simulink subsystem "BalanceLimit"  (R2023b)
settings: Solver=VariableStepAuto  StartTime=0.0  StopTime=10.0  RelTol=1e-3
libraries: simulink x1
settings Model: Creator=Veimar  LastModifiedBy=Veimar

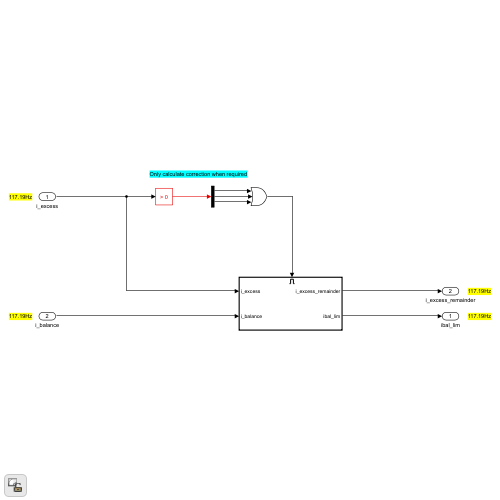
[thumbnail: Simulink's stored preview of the top-level diagram]
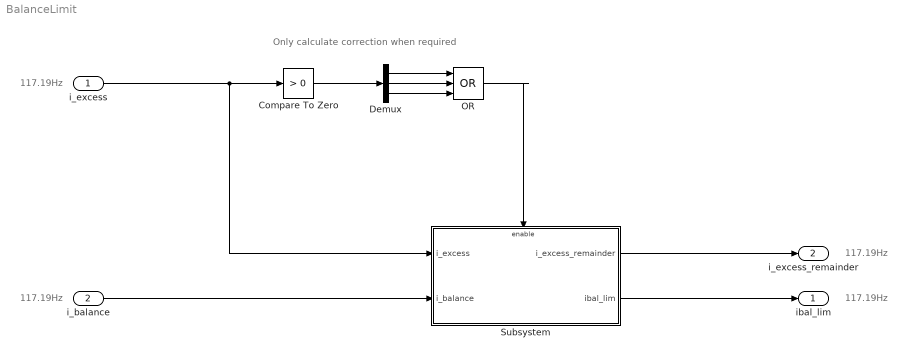
== system BalanceLimit ==
  note: Only calculate correction when required
  note: 117.19Hz
  note: 117.19Hz
  note: 117.19Hz
  note: 117.19Hz
  i_excess : Inport  OutDataTypeStr=single  PortDimensions=3
  i_balance : Inport  Port=2  OutDataTypeStr=single  PortDimensions=3
  Compare To Zero : simulink/Logic and Bit Operations/Compare To Zero  relop=>  OutDataTypeStr=boolean
  Demux : Demux  Outputs=3
  OR : Logic  Operator=OR  Inputs=3  IconShape=distinctive  AllPortsSameDT=off  OutDataTypeStr=boolean
  Subsystem : Subsystem
  ibal_lim : Outport  OutDataTypeStr=single  PortDimensions=3
  i_excess_remainder : Outport  Port=2  OutDataTypeStr=single  PortDimensions=3
  wires:
  OR/1 -> Subsystem/Enable
  Demux/3 -> OR/3
  Demux/2 -> OR/2
  Demux/1 -> OR/1
  Compare To Zero/1 -> Demux/1
  i_excess/1 -> Compare To Zero/1, Subsystem/1(i_excess)
  i_balance/1 -> Subsystem/2(i_balance)
  Subsystem/1(i_excess_remainder) -> i_excess_remainder/1
  Subsystem/2(ibal_lim) -> ibal_lim/1

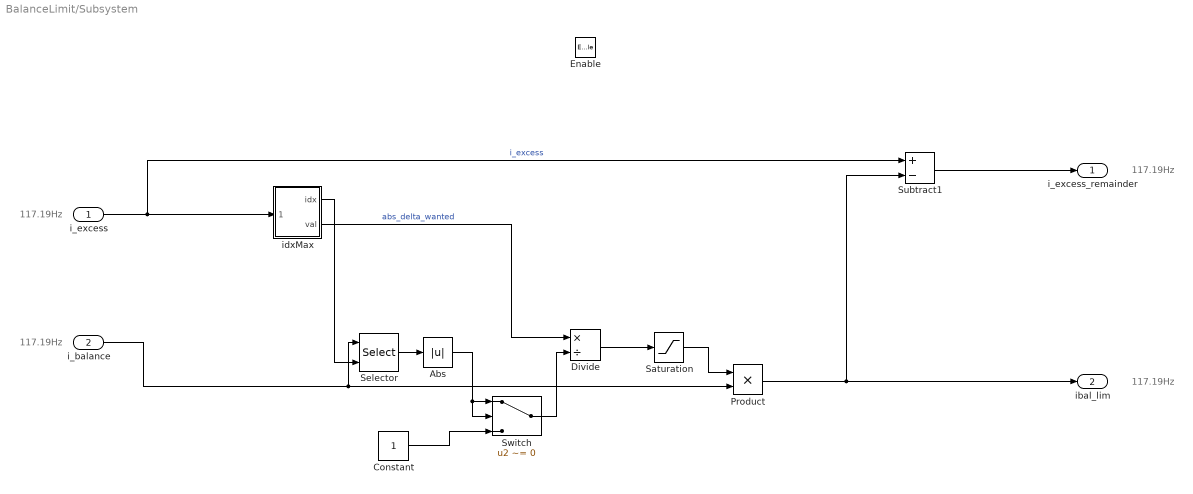
== system BalanceLimit/Subsystem ==
  note: 117.19Hz
  note: 117.19Hz
  note: 117.19Hz
  note: 117.19Hz
  i_excess : Inport
  i_balance : Inport  Port=2
  Enable : EnablePort  StatesWhenEnabling=reset
  Abs : Abs  SaturateOnIntegerOverflow=off
  Constant : Constant  OutDataTypeStr=single
  Divide : Product  Inputs=*/
  Product : Product
  Saturation : Saturate  UpperLimit=1  LowerLimit=0
  Selector : Selector  InputPortWidth=3  IndexOptions=Index vector (port)  Indices=[1 3]  OutputSizes=1
  Subtract1 : Sum  Inputs=+-
  Switch : Switch  Criteria=u2 ~= 0  SaturateOnIntegerOverflow=off  InputSameDT=off
  idxMax : Subsystem  mask(idxMinMax){maskOp=Max}
      mask prompts: maskOp "Operator"
      mask help:
      | <html><p>
      | The idxMinMax block determines the minimum or maximum value (as selected below)
      | of the input array and the corresponding index for that value. If there are
      | multiple instances of the min/max value, the index corresponds to the first one.
      | </p></html>
      mask TypeOptions maskOp: Min | Max
      mask Display: color('red');text(0.05,1,'Max','ver','top')
  i_excess_remainder : Outport  OutputWhenDisabled=reset  InitialOutput=0
  ibal_lim : Outport  Port=2  OutputWhenDisabled=reset  InitialOutput=0
  wires:
  Saturation/1 -> Product/1
  Divide/1 -> Saturation/1
  Abs/1 -> Switch/2, Switch/1
  idxMax/2(val) -> Divide/1  "abs_delta_wanted"
  Switch/1 -> Divide/2
  Selector/1 -> Abs/1
  Product/1 -> Subtract1/2, ibal_lim/1
  Constant/1 -> Switch/3
  idxMax/1(idx) -> Selector/2
  i_balance/1 -> Product/2, Selector/1
  i_excess/1 -> idxMax/1(array), Subtract1/1  "i_excess"
  Subtract1/1 -> i_excess_remainder/1

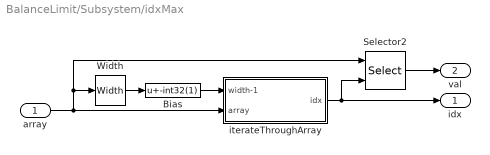
== system BalanceLimit/Subsystem/idxMax ==
  array : Inport
  Bias : Bias  Bias=-int32(1)  SaturateOnIntegerOverflow=off
  Selector2 : Selector  IndexOptions=Index vector (port)  Indices=[1 3]  OutputSizes=1
  Width : Width  DataType=int32
  iterateThroughArray : Subsystem
  idx : Outport
  val : Outport  Port=2
  wires:
  Selector2/1 -> val/1
  iterateThroughArray/1(idx) -> Selector2/2, idx/1
  Bias/1 -> iterateThroughArray/1(width-1)
  array/1 -> iterateThroughArray/2(array), Width/1, Selector2/1
  Width/1 -> Bias/1

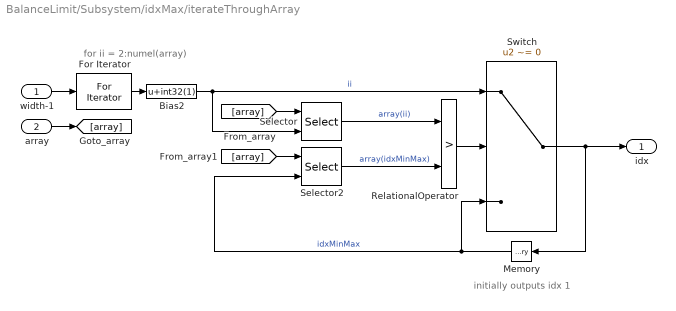
== system BalanceLimit/Subsystem/idxMax/iterateThroughArray ==
  note: for ii = 2:numel(array)
  note: initially outputs idx 1
  width-1 : Inport
  array : Inport  Port=2
  Bias2 : Bias  Bias=int32(1)  SaturateOnIntegerOverflow=off
  For Iterator : ForIterator  ResetStates=reset  IterationSource=external
  Memory : Memory  InitialCondition=int32(1)  InheritSampleTime=on
  RelationalOperator : RelationalOperator  Operator=>  OutDataTypeStr=boolean  InputSameDT=off
  Selector : Selector  IndexOptions=Index vector (port)  Indices=[1 3]  OutputSizes=1
  Selector2 : Selector  IndexOptions=Index vector (port)  Indices=[1 3]  OutputSizes=1
  Switch : Switch  Criteria=u2 ~= 0  SaturateOnIntegerOverflow=off  InputSameDT=off
  idx : Outport
  wires:
  Memory/1 -> Selector2/2, Switch/3  "idxMinMax"
  [array] -> Selector2/1
  Switch/1 -> idx/1, Memory/1
  array/1 -> [array]
  [array] -> Selector/1
  RelationalOperator/1 -> Switch/2
  Bias2/1 -> Selector/2, Switch/1  "ii"
  For Iterator/1 -> Bias2/1
  Selector2/1 -> RelationalOperator/2  "array(idxMinMax)"
  Selector/1 -> RelationalOperator/1  "array(ii)"
  width-1/1 -> For Iterator/1
